simulink model "PI_Controller"  (R2019b)
settings: Solver=VariableStepAuto  StartTime=0.0  StopTime=10.0  RelTol=1e-3
PreLoadFcn:
  | % parameter for PI_Controller
  | Kp=0.5;
  | Ki=0.5;
  | Ts=0.1;
settings Model: Creator=spuny  LastModifiedBy=spuny

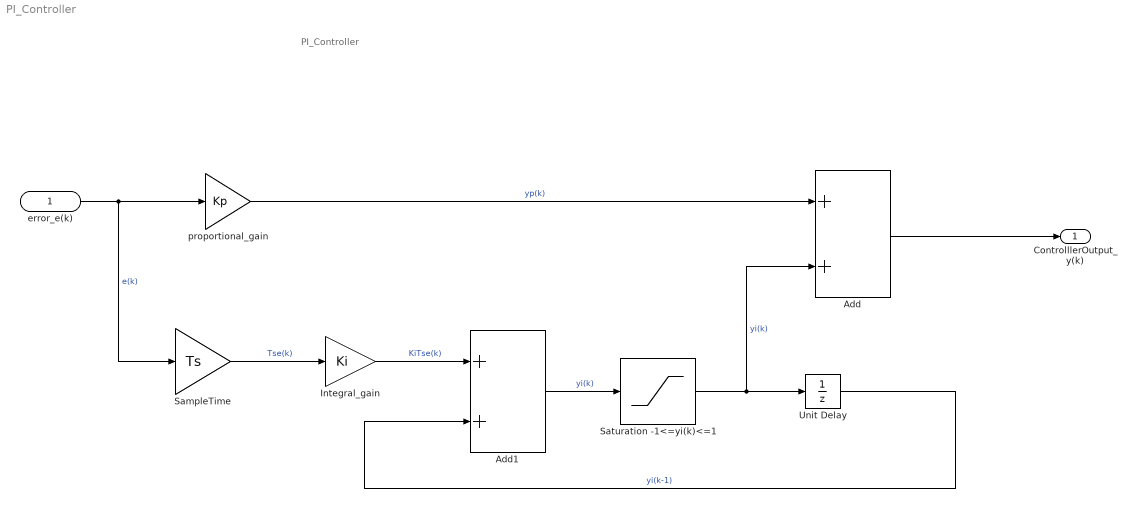
== system PI_Controller ==
  note: PI_Controller
  error_e(k) : Inport
  Add : Sum
  Add1 : Sum
  Integral_gain : Gain  Gain=Ki
  SampleTime : Gain  Gain=Ts
  Saturation -1<=yi(k)<=1 : Saturate  UpperLimit=+1  LowerLimit=-1
  Unit Delay : UnitDelay  SampleTime=Ts  HasFrameUpgradeWarning=on
  proportional_gain : Gain  Gain=Kp
  ControlllerOutput_y(k) : Outport
  wires:
  Add/1 -> ControlllerOutput_y(k)/1
  error_e(k)/1 -> SampleTime/1, proportional_gain/1  "e(k)"
  proportional_gain/1 -> Add/1  "yp(k)"
  SampleTime/1 -> Integral_gain/1  "Tse(k)"
  Integral_gain/1 -> Add1/1  "KiTse(k)"
  Add1/1 -> Saturation -1<=yi(k)<=1/1  "yi(k)"
  Saturation -1<=yi(k)<=1/1 -> Add/2, Unit Delay/1  "yi(k)"
  Unit Delay/1 -> Add1/2  "yi(k-1)"
